simulink model "LP7"  (R2021a)
settings: Solver=VariableStepAuto  StartTime=0.0  StopTime=10.0  RelTol=1e-3
undefined symbols (not defined in the file or in its folder): DiscIntNeverNeededParam
settings Model: Creator=Rubina  LastModifiedBy=Rubina

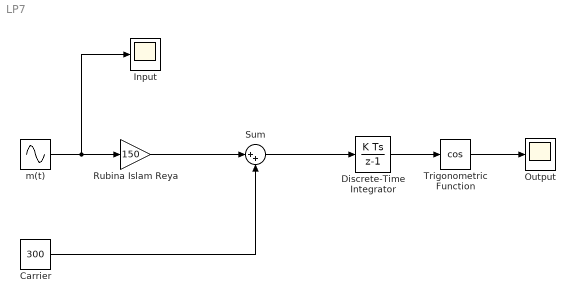
== system LP7 ==
  Carrier : Constant  Value=300
  Discrete-Time Integrator : DiscreteIntegrator  SampleTime=1/98000  ICPrevOutput=DiscIntNeverNeededParam  ICPrevScaledInput=DiscIntNeverNeededParam
  Input : Scope
  Output : Scope
  Rubina Islam Reya : Gain  Gain=150
  Sum : Sum  Inputs=|++
  Trigonometric Function : Trigonometry  Operator=cos
  m(t) : Sin  Frequency=10  Phase=90  SampleTime=1/98000
  wires:
  m(t)/1 -> Input/1, Rubina Islam Reya/1
  Rubina Islam Reya/1 -> Sum/1
  Carrier/1 -> Sum/2
  Sum/1 -> Discrete-Time Integrator/1
  Discrete-Time Integrator/1 -> Trigonometric Function/1
  Trigonometric Function/1 -> Output/1
